simulink library "tqd"  (R2021b)
settings: Solver=VariableStepAuto  StartTime=0.0  StopTime=10.0  RelTol=1e-3
undefined symbols (not defined in the file or in its folder): ATQD_APSDecReq_X_kph, ATQD_APSDecReq_Y_mps2, ATQD_APSDecReqCMD_X_kph, ATQD_APSDecReqTs_X_pct, ATQD_APSDecTimeGain_X_Deg, ATQD_APSDecTimeGain_Y_s, ATQD_APSReqLowSpd_X_Deg, ATQD_AutoHoldReleaseBPS_X_Deg, ATQD_AWDLoadTrqnsGain_X_kg, ATQD_AWDLoadTrqnsGain_Y_pct, ATQD_BOSEnBPSPosn_X_kph, ATQD_BOSMap_X_rpm, ATQD_BOSMap_Y_pct, ATQD_CreepBaseTqD_X_kph, ATQD_CreepBaseTqD_Y_Deg, ATQD_CreepBaseTqR_X_kph, ATQD_CreepBaseTqR_Y_Deg, ATQD_CreepBPSDisPosn_X_Deg, ATQD_CreepBPSDisPosnR_X_Deg, ATQD_CreepBPSEnPosn_X_Deg, ATQD_CreepBPSEnPosnR_X_Deg, ATQD_CreepDeltaTq_X_kph, ATQD_CreepIterm_X_kph, ATQD_CreepIterm_Y_kph, ATQD_CreepItermMaxLimit_X_pct, ATQD_CreepPreloadTime_X_kph, ATQD_CreepPreloadTq_X_kph, ATQD_CreepPreloadTq_Y_s, ATQD_CreepProtTq_X_Deg, ATQD_CreepPterm_X_kph, ATQD_CreepPterm_Y_kph, ATQD_ECOTqMapD_X_rpm, ATQD_ECOTqMapD_Y_pct, ATQD_EOPDTqMapDCon_X_rpm, ATQD_EOPDTqMapDCon_Y_Deg, ATQD_EstInitVehWeight_X_c, ATQD_LHMRollGenMapD_X_rpm, ATQD_LHMRollGenMapD_Y_rpm, ATQD_LHMTqMapD_X_rpm, ATQD_LHMTqMapD_Y_pct, ATQD_NL1TqMapD_X_rpm, ATQD_NL1TqMapD_Y_pct, ATQD_NOPDTqMapDCon_X_rpm, ATQD_NOPDTqMapDCon_Y_Deg, ATQD_NRMRrEDUSpRat_X_rpm, ATQD_NRMRrEDUSpRat_Y_Nm, ATQD_OPDHoldDownRelDelay_X_Deg, ATQD_OPDHoldEnSpd_X_Deg, ATQD_OPDHoldRelDetTime_X_Deg, ATQD_OPDHoldReleaseTq_X_Deg, ATQD_OrigPedTqLowLim_X_Deg, ATQD_OrigPedTqLowLim_Y_pct, ATQD_PedalMapClimbUpLim_X_rpm, ATQD_PedalMapClimbUpLim_Y_Deg, ATQD_PreLoadTq_X_s, ATQD_RollGenMapEL1_X_rpm, ATQD_RollGenMapEL1_Y_rpm, ATQD_SL1TqMapD_X_rpm, ATQD_SL1TqMapD_Y_pct, ATQD_SlideRegenTqGain_X_Gps ... (+491)
libraries: hcu_lib x83, simulink x73, tqr x1
(part 7 of 19)

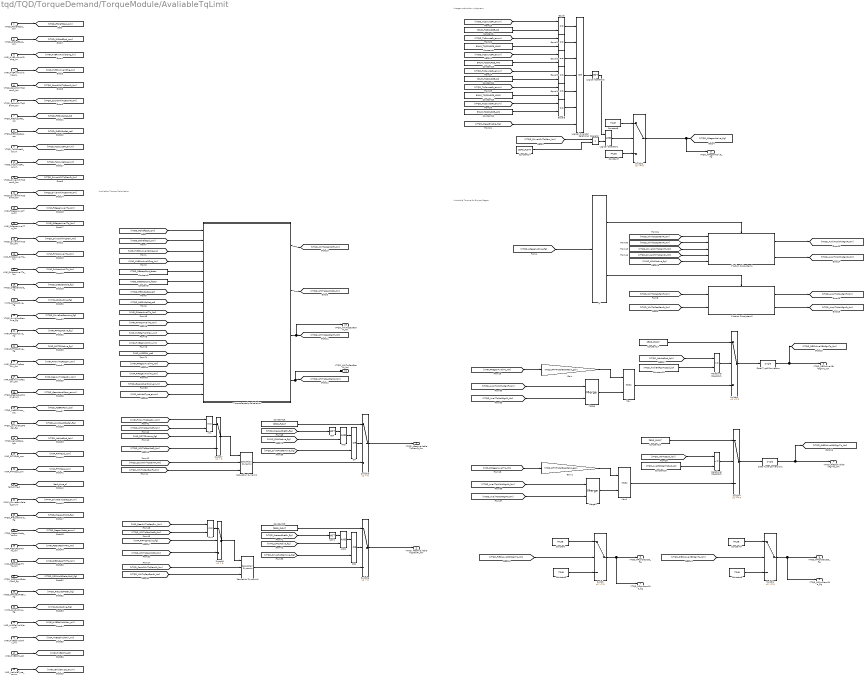
== system tqd/TQD/TorqueDemand/TorqueModule/AvaliableTqLimit ==
  note: Avaiable Torque for B-type Regen
  note: Available Torque Calculation
  note: A-regen activation judgment
  VTQD_FrShaftSpd_rpm : Inport
  VTQD_RrShaftSpd_rpm : Inport  Port=2
  VINP_HVBPwrAvailDchrg_kw : Inport  Port=3
  VINP_HVBPwrAvailChrg_kw : Inport  Port=4
  VTQD_CoordWhlTqDemFr_Nm : Inport  Port=5
  VTQD_CoordWhlTqDemRr_Nm : Inport  Port=6
  VTQD_FrEDUSpRat_rat : Inport  Port=7
  VTQD_RrEDUSpRat_rat : Inport  Port=8
  VTQD_TqSourceFr_enum : Inport  Port=9
  VTQD_TqSourceRr_enum : Inport  Port=10
  VTQD_DriverWhlTqDemFr_Nm : Inport  Port=11
  VTQD_DriverWhlTqDemRr_Nm : Inport  Port=12
  VINP_FrRegenAvailTq_Nm : Inport  Port=13
  VINP_RrRegenAvailTq_Nm : Inport  Port=14
  VTQD_DriverWhlTqDem_Nm : Inport  Port=15
  VINP_FrMotorAvailTq_Nm : Inport  Port=16
  VINP_RrMotorAvailTq_Nm : Inport  Port=17
  VTQD_CreepEnable_flg : Inport  Port=18
  VVMC_ADASActive_flg : Inport  Port=19
  VTQD_DriveProtRemove_flg : Inport  Port=20
  VINP_FrPTCSActive_flg : Inport  Port=21
  VINP_RrPTCSActive_flg : Inport  Port=22
  VINP_FrntAxlTrqReqDrv_Nm : Inport  Port=23
  VINP_RearAxlTrqReqDrv_Nm : Inport  Port=24
  VTQD_GearActualPosn_enum : Inport  Port=25
  VTQD_ActBPSPosn_pct : Inport  Port=26
  VTQD_LowIdleAccPedal_flg : Inport  Port=27
  VTQD_VehActSpd_kph : Inport  Port=28
  VINP_RrTMSpd_rpm : Inport  Port=29
  VINP_FrTMSpd_rpm : Inport  Port=30
  task_time_s : Inport  Port=31
  VPMM_DrivetrainSelect_enum : Inport  Port=32
  VTQD_PreLoadHold_flg : Inport  Port=33
  VTQD_RegenMode_enum : Inport  Port=34
  VINP_FrEDURealTMTq_Nm : Inport  Port=35
  VINP_RrEDURealTMTq_Nm : Inport  Port=36
  VTQD_OPDHoldDelayForP_flg : Inport  Port=37
  VTQD_PreLoadPreEn_flg : Inport  Port=38
  VVMC_CAASActive_flg : Inport  Port=39
  VINP_HVBCellVoltMax_mV : Inport  Port=40
  VINP_HVBCellVoltMin_mV : Inport  Port=41
  VINP_HVBSOH_pct : Inport  Port=42
  VINP_VehicleType_enum : Inport  Port=43
  AND : Logic  AllPortsSameDT=off  OutDataTypeStr=boolean
  AND1 : Logic  AllPortsSameDT=off  OutDataTypeStr=boolean
  Constant : Constant  Value=FALSE
  Constant1 : Constant  Value=ENUM_TQSOURCE_CC
  Constant10 : Constant  Value=ENUM_TQSOURCE_APS
  Constant11 : Constant  Value=ENUM_TQSOURCE_CC
  Constant12 : Constant  Value=ENUM_TQSOURCE_APS
  Constant13 : Constant  Value=ENUM_TQSOURCE_ADAS
  Constant{14,16..17,19..20} (5 alike) : Constant  Value=ZERO_FLOAT
  Constant15 : Constant  Value=KTQD_AvailBrkRgnTqSpd_kph
  Constant18 : Constant  Value=KTQD_AvailBrkRgnTqSpd_kph
  Constant2 : Constant  Value=KTQD_FrBatapCont_factor
  Constant3 : Constant  Value=TRUE
  Constant4 : Constant  Value=FALSE
  Constant5 : Constant  Value=KTQD_RrBatapCont_factor
  Constant6 : Constant  Value=TRUE
  Constant7 : Constant  Value=FALSE
  Constant8 : Constant  Value=TRUE
  Constant9 : Constant  Value=ENUM_TQSOURCE_ADAS
  Data Type Conversion : DataTypeConversion  OutDataTypeStr=single
  Data Type Conversion1 : DataTypeConversion  OutDataTypeStr=single
  Equal{,1..5} (6 alike) : RelationalOperator  Operator===  OutDataTypeStr=boolean  RndMeth=Simplest
  Gain : Gain  Gain=KTQD_FrTMTotalGearRatio_gain
  Gain1 : Gain  Gain=KTQD_RrTMTotalGearRatio_gain
  If : If  IfExpression=u1 ~= 0
  If Action Subsystem1 : Subsystem  TreatAsAtomicUnit=on
  If Action Subsystem2 : Subsystem  TreatAsAtomicUnit=on
  Logical Operator : Logic  Operator=OR  Inputs=7  AllPortsSameDT=off  OutDataTypeStr=boolean
  Logical Operator1 : Logic  AllPortsSameDT=off  OutDataTypeStr=boolean
  Logical Operator2 : Logic  Operator=NOT  AllPortsSameDT=off  OutDataTypeStr=boolean
  Max : MinMax  Function=max  Inputs=2
  Max1 : MinMax  Function=max  Inputs=2
  Merge : Merge
  Merge1 : Merge
  Min : MinMax  Inputs=2
  Min1 : MinMax  Inputs=2
  NOT : Logic  Operator=NOT  AllPortsSameDT=off  OutDataTypeStr=boolean
  NOT1 : Logic  Operator=NOT  AllPortsSameDT=off  OutDataTypeStr=boolean
  OR : Logic  Operator=OR  AllPortsSameDT=off  OutDataTypeStr=boolean
  OR1 : Logic  Operator=OR  AllPortsSameDT=off  OutDataTypeStr=boolean
  Relational Operator : RelationalOperator  Operator=<  OutDataTypeStr=boolean  RndMeth=Simplest
  Relational Operator1 : RelationalOperator  Operator=<=  OutDataTypeStr=boolean  RndMeth=Simplest
  Relational Operator2 : RelationalOperator  Operator=<=  OutDataTypeStr=boolean  RndMeth=Simplest
  Saturation Dynamic : simulink/Discontinuities/Saturation Dynamic  OutMin=[]  OutMax=[]  OutDataTypeStr=Inherit: Same as second input  OutDataType=fixdt(1, 16)  OutScaling=2^-10  DoSatur=off
  Saturation Dynamic1 : simulink/Discontinuities/Saturation Dynamic  OutMin=[]  OutMax=[]  OutDataTypeStr=Inherit: Same as second input  OutDataType=fixdt(1, 16)  OutScaling=2^-10  DoSatur=off
  Switch : Switch
  Switch1 : Switch
  Switch2 : Switch  Criteria=u2 ~= 0
  Switch3 : Switch  Criteria=u2 ~= 0
  Switch4 : Switch  Criteria=u2 ~= 0
  Switch{5..8} (4 alike) : Switch  Criteria=u2 > Threshold
  TorqueCapacityCalcalation : Subsystem
  VTQD_AfterAvailableTqDemFr_Nm : Outport
  VTQD_AfterAvailableTqDemRr_Nm : Outport  Port=2
  VTQD_FrEDUAvailBrkRgnTq_Nm : Outport  Port=3
  VTQD_RrEDUAvailBrkRgnTq_Nm : Outport  Port=4
  VTQD_FrRgnDecrSta_flg : Outport  Port=5
  VTQD_RrRgnDecrSta_flg : Outport  Port=6
  VTQD_FrRgnPermSta_flg : Outport  Port=7
  VTQD_RrRgnPermSta_flg : Outport  Port=8
  VTQD_ARegenActive_flg : Outport  Port=9
  VTQD_WhlTqCapGenFr_Nm : Outport  Port=10
  VTQD_WhlTqCapGenRr_Nm : Outport  Port=11
  wires:
  VINP_FrRegenAvailTq_Nm/1 -> [VINP_FrRegenAvailTq_Nm]
  VINP_RrRegenAvailTq_Nm/1 -> [VINP_RrRegenAvailTq_Nm]
  Merge1/1 -> Max1/2
  [VINP_RrRegenAvailTq_Nm] -> Gain1/1
  Gain1/1 -> Max1/1
  Gain/1 -> Max/1
  Merge/1 -> Max/2
  [VINP_FrRegenAvailTq_Nm] -> Gain/1
  [VTQD_ARegenActive_flg] -> If/1
  Switch1/1 -> VTQD_RrRgnDecrSta_flg/1, VTQD_RrRgnPermSta_flg/1
  Constant6/1 -> Switch1/3
  Constant4/1 -> Switch1/1
  [VTQD_RrEDUAvailBrkRgnTq_Nm] -> Switch1/2
  Switch/1 -> VTQD_FrRgnDecrSta_flg/1, VTQD_FrRgnPermSta_flg/1
  Constant3/1 -> Switch/3
  Constant/1 -> Switch/1
  [VTQD_FrEDUAvailBrkRgnTq_Nm] -> Switch/2
  If/2 -> If Action Subsystem2/Action
  If/1 -> If Action Subsystem1/Action
  Data Type Conversion1/1 -> VTQD_RrEDUAvailBrkRgnTq_Nm/1, [VTQD_RrEDUAvailBrkRgnTq_Nm]  "VTQD_RrEDUAvailBrkRgnTq_Nm"
  Data Type Conversion/1 -> VTQD_FrEDUAvailBrkRgnTq_Nm/1, [VTQD_FrEDUAvailBrkRgnTq_Nm]  "VTQD_FrEDUAvailBrkRgnTq_Nm"
  TorqueCapacityCalcalation/4(VTQD_WhlTqCapGenRr_Nm) -> VTQD_WhlTqCapGenRr_Nm/1, [VTQD_WhlTqCapGenRr_Nm]
  TorqueCapacityCalcalation/2(VTQD_WhlTqCapMotRr_Nm) -> [VTQD_WhlTqCapMotRr_Nm]
  VTQD_RrShaftSpd_rpm/1 -> [VTQD_RrShaftSpd_rpm]
  [VTQD_RrEDUSpRat_rat] -> TorqueCapacityCalcalation/8(VTQD_RrEDUSpRat_rat)
  [VTQD_FrEDUSpRat_rat] -> TorqueCapacityCalcalation/7(VTQD_FrEDUSpRat_cmd)
  Constant5/1 -> TorqueCapacityCalcalation/6(KTQD_RrBatapCont_factor)
  [VTQD_RrShaftSpd_rpm] -> TorqueCapacityCalcalation/2(VTQD_RrShaftSpd_rpm)
  Constant2/1 -> TorqueCapacityCalcalation/5(KTQD_FrBatapCont_factor)
  [VINP_HVBPwrAvailChrg_kw] -> TorqueCapacityCalcalation/4(VINP_HVBPwrAvailChrg_kw)
  [VINP_HVBPwrAvailDchrg_kw] -> TorqueCapacityCalcalation/3(VINP_HVBPwrAvailDchrg_kw)
  [VTQD_FrShaftSpd_rpm] -> TorqueCapacityCalcalation/1(VTQD_FrShaftSpd_rpm)
  TorqueCapacityCalcalation/1(VTQD_WhlTqCapMotFr_Nm) -> [VTQD_WhlTqCapMotFr_Nm]
  TorqueCapacityCalcalation/3(VTQD_WhlTqCapGenFr_Nm) -> VTQD_WhlTqCapGenFr_Nm/1, [VTQD_WhlTqCapGenFr_Nm]
  If Action Subsystem2/2(VTQD_AvailTqNoARgnRr_Nm) -> [VTQD_AvailTqNoARgnRr_Nm]
  If Action Subsystem2/1(VTQD_AvailTqNoARgnFr_Nm) -> [VTQD_AvailTqNoARgnFr_Nm]
  [VTQD_WhlTqCapGenRr_Nm] -> If Action Subsystem2/2(VTQD_WhlTqCapGenR_Nm)
  [VTQD_WhlTqCapGenFr_Nm] -> If Action Subsystem2/1(VTQD_WhlTqCapGenF_Nm)
  [VTQD_WhlTqCapGenRr_Nm] -> If Action Subsystem1/2(VTQD_WhlTqCapGenR_Nm)
  [VTQD_WhlTqCapGenFr_Nm] -> If Action Subsystem1/1(VTQD_WhlTqCapGenF_Nm)
  [VTQD_DriverWhlTqDemRr_Nm] -> If Action Subsystem1/4(VTQD_DriverWhlTqDemRr_Nm)
  [VTQD_DriverWhlTqDemFr_Nm] -> If Action Subsystem1/3(VTQD_DriverWhlTqDemFr_Nm)
  VTQD_DriverWhlTqDemRr_Nm/1 -> [VTQD_DriverWhlTqDemRr_Nm]
  VTQD_DriverWhlTqDemFr_Nm/1 -> [VTQD_DriverWhlTqDemFr_Nm]
  VTQD_TqSourceFr_enum/1 -> [VTQD_TqSourceFr_enum]
  VTQD_RrEDUSpRat_rat/1 -> [VTQD_RrEDUSpRat_rat]
  VTQD_FrEDUSpRat_rat/1 -> [VTQD_FrEDUSpRat_rat]
  VTQD_CoordWhlTqDemRr_Nm/1 -> [VTQD_CoordWhlTqDemRr_Nm]
  VTQD_CoordWhlTqDemFr_Nm/1 -> [VTQD_CoordWhlTqDemFr_Nm]
  VINP_HVBPwrAvailDchrg_kw/1 -> [VINP_HVBPwrAvailDchrg_kw]
  VTQD_FrShaftSpd_rpm/1 -> [VTQD_FrShaftSpd_rpm]
  VINP_HVBPwrAvailChrg_kw/1 -> [VINP_HVBPwrAvailChrg_kw]
  VTQD_TqSourceRr_enum/1 -> [VTQD_TqSourceRr_enum]
  Switch2/1 -> [VTQD_ARegenActive_flg], VTQD_ARegenActive_flg/1  "VTQD_ARegenActive_flg"
  VTQD_DriverWhlTqDem_Nm/1 -> [VTQD_DriverWhlTqDem_Nm]
  VINP_RrMotorAvailTq_Nm/1 -> [VINP_RrMotorAvailTq_Nm]
  VINP_FrMotorAvailTq_Nm/1 -> [VINP_FrMotorAvailTq_Nm]
  [VINP_FrMotorAvailTq_Nm] -> TorqueCapacityCalcalation/9(VINP_FrMotorAvailTq_Nm)
  [VINP_RrMotorAvailTq_Nm] -> TorqueCapacityCalcalation/10(VINP_RrMotorAvailTq_Nm)
  VTQD_CreepEnable_flg/1 -> [VTQD_CreepEnable_flg]
  [VTQD_TqSourceFr_enum] -> Equal/1
  Constant1/1 -> Equal/2
  Constant9/1 -> Equal1/2
  [VTQD_TqSourceFr_enum] -> Equal1/1
  [VTQD_TqSourceFr_enum] -> Equal2/1
  Constant10/1 -> Equal2/2
  Constant12/1 -> Equal5/2
  [VTQD_TqSourceRr_enum] -> Equal5/1
  [VTQD_TqSourceRr_enum] -> Equal4/1
  Constant13/1 -> Equal4/2
  Constant11/1 -> Equal3/2
  [VTQD_TqSourceRr_enum] -> Equal3/1
  Equal5/1 -> Logical Operator/6
  Equal4/1 -> Logical Operator/5
  Equal3/1 -> Logical Operator/4
  Equal2/1 -> Logical Operator/3
  Equal1/1 -> Logical Operator/2
  Equal/1 -> Logical Operator/1
  [VTQD_CreepEnable_flg] -> Logical Operator/7
  Logical Operator/1 -> Logical Operator2/1
  Logical Operator1/1 -> Switch2/2
  [VTQD_DriverWhlTqDem_Nm] -> Relational Operator/1
  Relational Operator/1 -> Logical Operator1/2
  Constant14/1 -> Relational Operator/2
  Constant7/1 -> Switch2/3
  Constant8/1 -> Switch2/1
  Logical Operator2/1 -> Logical Operator1/1
  Constant17/1 -> Switch3/1
  Relational Operator1/1 -> Switch3/2
  Constant15/1 -> Relational Operator1/2
  Max/1 -> Switch3/3
  Switch3/1 -> Data Type Conversion/1
  Constant20/1 -> Switch4/1
  Max1/1 -> Switch4/3
  Relational Operator2/1 -> Switch4/2
  Constant18/1 -> Relational Operator2/2
  Switch4/1 -> Data Type Conversion1/1
  VVMC_ADASActive_flg/1 -> [VVMC_ADASActive_flg]
  [VVMC_ADASActive_flg] -> If Action Subsystem1/5(VVMC_ADASActive_flg)
  [VTQD_AvailTqNoARgnRr_Nm] -> Merge1/2
  [VTQD_AvailTqWithARgnRr_Nm] -> Merge1/1
  [VTQD_AvailTqNoARgnFr_Nm] -> Merge/2
  [VTQD_AvailTqWithARgnFr_Nm] -> Merge/1
  Constant16/1 -> Switch5/1
  Switch5/1 -> VTQD_AfterAvailableTqDemFr_Nm/1  "VTQD_AfterAvailableTqDemFr_Nm"
  Saturation Dynamic/1 -> Switch5/3
  Constant19/1 -> Switch6/1
  Saturation Dynamic1/1 -> Switch6/3
  Switch6/1 -> VTQD_AfterAvailableTqDemRr_Nm/1  "VTQD_AfterAvailableTqDemRr_Nm"
  VTQD_DriveProtRemove_flg/1 -> [VTQD_DriveProtRemove_flg]
  [VTQD_CoordWhlTqDemFr_Nm] -> Saturation Dynamic/2
  Switch7/1 -> Saturation Dynamic/1  "VTQD_FrAvailableTqUpLimt_Nm"
  [VTQD_WhlTqCapMotFr_Nm] -> Switch7/3
  [VINP_FrPTCSActive_flg] -> Switch7/2
  VINP_RearAxlTrqReqDrv_Nm/1 -> [VINP_RearAxlTrqReqDrv_Nm]
  VINP_FrntAxlTrqReqDrv_Nm/1 -> [VINP_FrntAxlTrqReqDrv_Nm]
  VINP_RrPTCSActive_flg/1 -> [VINP_RrPTCSActive_flg]
  VINP_FrPTCSActive_flg/1 -> [VINP_FrPTCSActive_flg]
  [VINP_RrPTCSActive_flg] -> Switch8/2
  [VTQD_WhlTqCapMotRr_Nm] -> Switch8/3
  Switch8/1 -> Saturation Dynamic1/1  "VTQD_RrAvailableTqUpLimt_Nm"
  [VTQD_CoordWhlTqDemRr_Nm] -> Saturation Dynamic1/2
  [VTQD_WhlTqCapMotFr_Nm] -> Min/2
  Min/1 -> Switch7/1
  [VINP_FrntAxlTrqReqDrv_Nm] -> Min/1
  [VTQD_WhlTqCapMotRr_Nm] -> Min1/2
  Min1/1 -> Switch8/1
  [VINP_RearAxlTrqReqDrv_Nm] -> Min1/1
  VTQD_GearActualPosn_enum/1 -> [VTQD_GearActualPosn_enum]
  VTQD_ActBPSPosn_pct/1 -> [VTQD_ActBPSPosn_pct]
  VTQD_LowIdleAccPedal_flg/1 -> [VTQD_LowIdleAccPedal_flg]
  VTQD_VehActSpd_kph/1 -> [VTQD_VehActSpd_kph]
  VINP_RrTMSpd_rpm/1 -> [VINP_RrTMSpd_rpm]
  VINP_FrTMSpd_rpm/1 -> [VINP_FrTMSpd_rpm]
  task_time_s/1 -> [task_time_s]
  VPMM_DrivetrainSelect_enum/1 -> [VPMM_DrivetrainSelect_enum]
  [VTQD_VehActSpd_kph] -> Relational Operator1/1
  [VTQD_VehActSpd_kph] -> Relational Operator2/1
  [VTQD_WhlTqCapGenFr_Nm] -> Saturation Dynamic/3
  [VTQD_WhlTqCapGenRr_Nm] -> Saturation Dynamic1/3
  VTQD_PreLoadHold_flg/1 -> [VTQD_PreLoadHold_flg]
  VTQD_RegenMode_enum/1 -> [VTQD_RegenMode_enum]
  VINP_RrEDURealTMTq_Nm/1 -> [VINP_RrEDURealTMTq_Nm]
  VINP_FrEDURealTMTq_Nm/1 -> [VINP_FrEDURealTMTq_Nm]
  VTQD_OPDHoldDelayForP_flg/1 -> [VTQD_OPDHoldDelayForP_flg]
  VVMC_CAASActive_flg/1 -> [VVMC_CAASActive_flg]
  VTQD_PreLoadPreEn_flg/1 -> [VTQD_PreLoadPreEn_flg]
  OR/1 -> Switch5/2
  AND/1 -> OR/1
  [VTQD_DriveProtRemove_flg] -> OR/2
  NOT/1 -> AND/1
  [VTQD_PreLoadPreEn_flg] -> NOT/1
  [VVMC_CAASActive_flg] -> AND/2
  NOT1/1 -> AND1/1
  AND1/1 -> OR1/1
  [VVMC_CAASActive_flg] -> AND1/2
  [VTQD_PreLoadPreEn_flg] -> NOT1/1
  [VTQD_DriveProtRemove_flg] -> OR1/2
  OR1/1 -> Switch6/2
  VINP_HVBCellVoltMin_mV/1 -> [VINP_HVBCellVoltMin_mV]
  VINP_HVBSOH_pct/1 -> [VINP_HVBSOH_pct]
  VINP_HVBCellVoltMax_mV/1 -> [VINP_HVBCellVoltMax_mV]
  [VINP_HVBCellVoltMax_mV] -> TorqueCapacityCalcalation/11(VINP_HVBCellVoltMax_mV)
  [VINP_HVBCellVoltMin_mV] -> TorqueCapacityCalcalation/12(VINP_HVBCellVoltMin_mV)
  [VINP_HVBSOH_pct] -> TorqueCapacityCalcalation/13(VINP_HVBSOH_pct)
  If Action Subsystem1/1(VTQD_AvailTqWithARgnFr_Nm) -> [VTQD_AvailTqWithARgnFr_Nm]
  If Action Subsystem1/2(VTQD_AvailTqWithARgnRr_Nm) -> [VTQD_AvailTqWithARgnRr_Nm]
  [VINP_RrRegenAvailTq_Nm] -> TorqueCapacityCalcalation/15(VINP_RrRegenAvailTq_Nm)
  [VINP_FrRegenAvailTq_Nm] -> TorqueCapacityCalcalation/14(VINP_FrRegenAvailTq_Nm)
  [VTQD_GearActualPosn_enum] -> TorqueCapacityCalcalation/16(VTQD_GearActualPosn_enum)
  VINP_VehicleType_enum/1 -> [VINP_VehicleType_enum]
  [VINP_VehicleType_enum] -> TorqueCapacityCalcalation/17(VINP_VehicleType_enum)

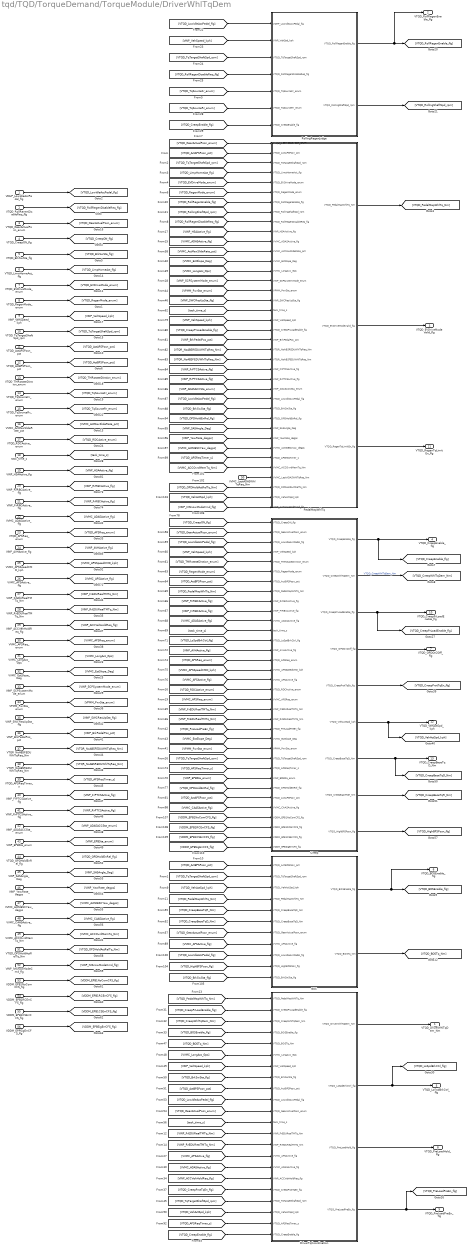
== system tqd/TQD/TorqueDemand/TorqueModule/DriverWhlTqDem ==
  VDHP_LowIdleAccPedal_flg : Inport
  VTQD_RollRegenDisableReq_flg : Inport  Port=2
  VTQD_GearActualPosn_enum : Inport  Port=3
  "VTQD_CreepON_flg " : Inport  Port=4
  VTQD_BrkSwSta_flg : Inport  Port=5
  VTQD_LimpHomeAct_flg : Inport  Port=6
  VTQD_EVDriveMode_enum : Inport  Port=7
  VTQD_RegenMode_enum : Inport  Port=8
  VINP_VehSpeed_kph : Inport  Port=9
  VTQD_TqTargetShaftSpd_rpm : Inport  Port=10
  VTQD_ActAPSPosn_pct : Inport  Port=11
  VTQD_ActBPSPosn_pct : Inport  Port=12
  VTQD_TMRotateDirction_enum : Inport  Port=13
  VTQD_TqSourceFr_enum : Inport  Port=14
  VTQD_TqSourceRr_enum : Inport  Port=15
  VVMC_ActMaxSlideRate_pct : Inport  Port=16
  VTQD_RDCActive_enum : Inport  Port=17
  task_time_s : Inport  Port=18
  VINP_HSAActive_flg : Inport  Port=19
  VINP_RrRBCActive_flg : Inport  Port=20
  VINP_FrRBCActive_flg : Inport  Port=21
  VVMC_ADASActive_flg : Inport  Port=22
  VTQD_APSReq_enum : Inport  Port=23
  VINP_AVHActive_flg : Inport  Port=24
  VVMC_APSSpeedCMD_kph : Inport  Port=25
  VVMC_APSActive_flg : Inport  Port=26
  VINP_FrEDURealTMTq_Nm : Inport  Port=27
  VINP_RrEDURealTMTq_Nm : Inport  Port=28
  VINP_ACCVehHoldReq_flg : Inport  Port=29
  VVMC_APSReq_enum : Inport  Port=30
  VVMC_LongAcc_Gps : Inport  Port=31
  VVMC_EstSlope_Deg : Inport  Port=32
  VINP_SCPSystemMode_enum : Inport  Port=33
  VPMM_PwrSta_enum : Inport  Port=34
  VINP_SWCResUpSta_flg : Inport  Port=35
  VINP_BrkPedalPos_pct : Inport  Port=36
  VTQR_NoABSFEDUWhlTqReq_Nm : Inport  Port=37
  VTQR_NoABSREDUWhlTqReq_Nm : Inport  Port=38
  VTQD_APSReqTimer_s : Inport  Port=39
  VINP_FrPTCSActive_flg : Inport  Port=40
  VINP_RrPTCSActive_flg : Inport  Port=41
  VINP_ADASACCSta_enum : Inport  Port=42
  VINP_EPBSta_enum : Inport  Port=43
  VTQD_OPDHoldEnRel_flg : Inport  Port=44
  VINP_SASAngle_Deg : Inport  Port=45
  VINP_YawRate_degps : Inport  Port=46
  VVMC_ActStESCYaw_degps : Inport  Port=47
  VVMC_CAASActive_flg : Inport  Port=48
  VVMC_ACCOvrdMemTq_Nm : Inport  Port=49
  VVMC_LastADASWhlTqReq_Nm : Inport  Port=50
  VTQD_OPDHoldActRelTq_Nm : Inport  Port=51
  VINP_IVISnowModeCmd_flg : Inport  Port=52
  VDDM_EPB1NoComCFS_flg : Inport  Port=53
  VDDM_EPB1RCErrCFS_flg : Inport  Port=54
  VDDM_EPB1CSErrCFS_flg : Inport  Port=55
  VDDM_EPBSigErrCFS_flg : Inport  Port=56
  BOS : Subsystem
  Creep : Subsystem
  DriverTqCoordination : Subsystem
  PedalMapWhlTq : Subsystem
  RollingRegenJudge : Subsystem
  VTQD_DriverWhlTqDem_Nm : Outport
  VTQD_RollRegenEnable_flg : Outport  Port=2
  VTQD_EVDriveModeValid_flg : Outport  Port=3
  VTQD_CreepEnable_flg : Outport  Port=4
  VTQD_LoSpdBrkCtrl_flg : Outport  Port=5
  VTQD_BOSEnable_flg : Outport  Port=6
  VTQD_OPDOn2Off_flg : Outport  Port=7
  VTQD_PreLoadHold_flg : Outport  Port=8
  VTQD_PreLoadPreEn_flg : Outport  Port=9
  VTQD_CreepPrLoadEnable_flg : Outport  Port=10
  VTQD_RegenTqLimitEn_flg : Outport  Port=11
  VTQD_VehActSpd_kph : Outport  Port=12
  VTQD_CreepBaseTqD_Nm : Outport  Port=13
  wires:
  VTQD_BrkSwSta_flg/1 -> [VTQD_BrkSwSta_flg]
  VTQD_ActBPSPosn_pct/1 -> [VTQD_ActBPSPosn_pct]
  VTQD_RegenMode_enum/1 -> [VTQD_RegenMode_enum]
  VINP_VehSpeed_kph/1 -> [VINP_VehSpeed_kph]
  "VTQD_CreepON_flg "/1 -> [VTQD_CreepON_flg]
  PedalMapWhlTq/1(VTQD_PedalMapWhlTq_Nm) -> [VTQD_PedalMapWhlTq_Nm]
  VTQD_LimpHomeAct_flg/1 -> [VTQD_LimpHomeAct_flg]
  VTQD_TqTargetShaftSpd_rpm/1 -> [VTQD_TqTargetShaftSpd_rpm]
  VTQD_EVDriveMode_enum/1 -> [VTQD_EVDriveMode_enum]
  VTQD_ActAPSPosn_pct/1 -> [VTQD_ActAPSPosn_pct]
  VTQD_GearActualPosn_enum/1 -> [VTQD_GearActualPosn_enum]
  VDHP_LowIdleAccPedal_flg/1 -> [VTQD_LowIdleAccPedal_flg]
  BOS/2(VTQD_BOSTq_Nm) -> [VTQD_BOSTq_Nm]
  BOS/1(VTQD_BOSEnable_flg) -> [VTQD_BOSEnable_flg], VTQD_BOSEnable_flg/1
  [VTQD_ActBPSPosn_pct] -> BOS/1(VTQD_ActBPSPosn_pct)
  [VTQD_TqTargetShaftSpd_rpm] -> BOS/2(VTQD_TqTargetShaftSpd_rpm)
  RollingRegenJudge/1(VTQD_RollRegenEnable_flg) -> VTQD_RollRegenEnable_flg/1, [VTQD_RollRegenEnable_flg]
  RollingRegenJudge/2(VTQD_RollingShaftSpd_rpm) -> [VTQD_RollingShaftSpd_rpm]
  VTQD_RollRegenDisableReq_flg/1 -> [VTQD_RollRegenDisableReq_flg]
  PedalMapWhlTq/2(VTQD_EVDriveModeValid_flg) -> VTQD_EVDriveModeValid_flg/1
  VTQD_TMRotateDirction_enum/1 -> [VTQD_TMRotateDirction_enum]
  [VTQD_GearActualPosn_enum] -> PedalMapWhlTq/1(VTQD_GearActualPosn_enum)
  [VTQD_LimpHomeAct_flg] -> PedalMapWhlTq/4(VTQD_LimpHomeAct_flg)
  [VTQD_ActAPSPosn_pct] -> PedalMapWhlTq/2(VTQD_ActAPSPosn_pct)
  [VTQD_TqTargetShaftSpd_rpm] -> PedalMapWhlTq/3(VTQD_TqTargetShaftSpd_rpm)
  [VTQD_RollRegenEnable_flg] -> PedalMapWhlTq/7(VTQD_RollRegenEnable_flg)
  [VTQD_RollingShaftSpd_rpm] -> PedalMapWhlTq/8(VTQD_RollingShaftSpd_rpm)
  [VTQD_RegenMode_enum] -> PedalMapWhlTq/6(VTQD_RegenMode_enum)
  [VTQD_EVDriveMode_enum] -> PedalMapWhlTq/5(VTQD_EVDriveMode_enum)
  [VTQD_TqSourceRr_enum] -> RollingRegenJudge/6(VTQD_TqSourceRr_enum)
  [VINP_VehSpeed_kph] -> RollingRegenJudge/2(VINP_VehSpd_kph)
  [VTQD_TqTargetShaftSpd_rpm] -> RollingRegenJudge/3(VTQD_TqTargetShaftSpd_rpm)
  [VTQD_TqSourceFr_enum] -> RollingRegenJudge/5(VTQD_TqSourceFr_enum)
  [VTQD_CreepEnable_flg] -> RollingRegenJudge/7(VTQD_CreepEnable_flg)
  [VTQD_LowIdleAccPedal_flg] -> RollingRegenJudge/1(VDHP_LowIdleAccPedal_flg)
  VTQD_TqSourceFr_enum/1 -> [VTQD_TqSourceFr_enum]
  VTQD_TqSourceRr_enum/1 -> [VTQD_TqSourceRr_enum]
  VVMC_ActMaxSlideRate_pct/1 -> [VVMC_ActMaxSlideRate_pct]
  VTQD_RDCActive_enum/1 -> [VTQD_RDCActive_enum]
  task_time_s/1 -> [task_time_s]
  [VTQD_RollRegenDisableReq_flg] -> RollingRegenJudge/4(VTQD_RollRegenDisableReq_flg)
  [VINP_VehSpeed_kph] -> DriverTqCoordination/7(VINP_VehSpeed_kph)
  [task_time_s] -> DriverTqCoordination/12(task_time_s)
  [VTQD_LowIdleAccPedal_flg] -> DriverTqCoordination/10(VTQD_LowIdleAccPedal_flg)
  [VTQD_GearActualPosn_enum] -> DriverTqCoordination/11(VTQD_GearActualPosn_enum)
  [VTQD_CreepPrLoadEnable_flg] -> DriverTqCoordination/2(VTQD_CreepPrLoadEnable_flg)
  [VTQD_PedalMapWhlTq_Nm] -> DriverTqCoordination/1(VTQD_PedalMapWhlTq_Nm)
  [VTQD_ActBPSPosn_pct] -> DriverTqCoordination/9(VTQD_ActBPSPosn_pct)
  [VTQD_BOSEnable_flg] -> DriverTqCoordination/4(VTQD_BOSEnable_flg)
  [VTQD_CreepWhlTqDem_Nm] -> DriverTqCoordination/3(VTQD_CreepWhlTqDem_Nm)
  [VTQD_BrkSwSta_flg] -> DriverTqCoordination/8(VTQD_BrkSwSta_flg)
  DriverTqCoordination/2(VTQD_LoSpdBrkCtrl_flg) -> [VTQD_LoSpdBrkCtrl_flg], VTQD_LoSpdBrkCtrl_flg/1
  DriverTqCoordination/1(VTQD_DriverWhlTqDem_Nm) -> VTQD_DriverWhlTqDem_Nm/1
  [VINP_RrRBCActive_flg] -> Creep/9(VINP_RrRBCActive_flg)
  [VINP_FrRBCActive_flg] -> Creep/10(VINP_FrRBCActive_flg)
  [VINP_VehSpeed_kph] -> Creep/4(VINP_VehSpeed_kph)
  [VTQD_ActBPSPosn_pct] -> Creep/7(VTQD_ActBPSPosn_pct)
  [VTQD_TMRotateDirction_enum] -> Creep/5(VTQD_TMRotateDirction_enum)
  [VTQD_CreepON_flg] -> Creep/1(VTQD_CreepON_flg)
  [VTQD_LowIdleAccPedal_flg] -> Creep/3(VTQD_LowIdleAccPedal_flg)
  [VTQD_APSReq_enum] -> Creep/15(VTQD_APSReq_enum)
  [VVMC_APSActive_flg] -> Creep/17(VVMC_APSActive_flg)
  [VTQD_RegenMode_enum] -> Creep/6(VTQD_RegenMode_enum)
  [VINP_AVHActive_flg] -> Creep/14(VINP_AVHActive_flg)
  [VVMC_APSSpeedCMD_kph] -> Creep/16(VVMC_APSSpeedCMD_kph)
  [VTQD_PedalMapWhlTq_Nm] -> Creep/8(VTQD_PedalMapWhlTq_Nm)
  [VTQD_GearActualPosn_enum] -> Creep/2(VTQD_GearActualPosn_enum)
  [VVMC_ADASActive_flg] -> Creep/11(VVMC_ADASActive_flg)
  [task_time_s] -> Creep/12(task_time_s)
  [VTQD_LoSpdBrkCtrl_flg] -> Creep/13(VTQD_LoSpdBrkCtrl_flg)
  Creep/1(VTQD_CreepEnable_flg) -> [VTQD_CreepEnable_flg], VTQD_CreepEnable_flg/1
  Creep/2(VTQD_CreepWhlTqDem_Nm) -> [VTQD_CreepWhlTqDem_Nm]  "VTQD_CreepWhlTqDem_Nm"
  Creep/3(VTQD_CreepPrLoadEnable_flg) -> VTQD_CreepPrLoadEnable_flg/1, [VTQD_CreepPrLoadEnable_flg]
  VVMC_APSActive_flg/1 -> [VVMC_APSActive_flg]
  VTQD_APSReq_enum/1 -> [VTQD_APSReq_enum]
  VVMC_ADASActive_flg/1 -> [VVMC_ADASActive_flg]
  VINP_AVHActive_flg/1 -> [VINP_AVHActive_flg]
  VVMC_APSSpeedCMD_kph/1 -> [VVMC_APSSpeedCMD_kph]
  VINP_FrRBCActive_flg/1 -> [VINP_FrRBCActive_flg]
  VINP_RrRBCActive_flg/1 -> [VINP_RrRBCActive_flg]
  VINP_HSAActive_flg/1 -> [VINP_HSAActive_flg]
  [VTQD_RollRegenDisableReq_flg] -> PedalMapWhlTq/9(VTQD_RollRegenDisableReq_flg)
  [VINP_HSAActive_flg] -> PedalMapWhlTq/10(VINP_HSAActive_flg)
  Creep/4(VTQD_OPDOn2Off_flg) -> VTQD_OPDOn2Off_flg/1
  VINP_RrEDURealTMTq_Nm/1 -> [VINP_RrEDURealTMTq_Nm]
  VINP_FrEDURealTMTq_Nm/1 -> [VINP_FrEDURealTMTq_Nm]
  [VINP_FrEDURealTMTq_Nm] -> DriverTqCoordination/13(VINP_FrEDURealTMTq_Nm)
  [VINP_RrEDURealTMTq_Nm] -> DriverTqCoordination/14(VINP_RrEDURealTMTq_Nm)
  DriverTqCoordination/3(VTQD_PreLoadHold_flg) -> VTQD_PreLoadHold_flg/1
  [VVMC_ADASActive_flg] -> PedalMapWhlTq/11(VVMC_ADASActive_flg)
  [VTQD_RDCActive_enum] -> Creep/18(VTQD_RDCActive_enum)
  VINP_ACCVehHoldReq_flg/1 -> [VINP_ACCVehHoldReq_flg]
  VVMC_APSReq_enum/1 -> [VVMC_APSReq_enum]
  [VVMC_APSReq_enum] -> Creep/19(VVMC_APSReq_enum)
  [VVMC_APSActive_flg] -> DriverTqCoordination/15(VVMC_APSActive_flg)
  [VVMC_ADASActive_flg] -> DriverTqCoordination/16(VVMC_ADASActive_flg)
  [VINP_ACCVehHoldReq_flg] -> DriverTqCoordination/17(VINP_ACCVehHoldReq_flg)
  [VINP_RrEDURealTMTq_Nm] -> Creep/21(VINP_RrEDURealTMTq_Nm)
  [VINP_FrEDURealTMTq_Nm] -> Creep/20(" VINP_FrEDURealTMTq_Nm")
  Creep/5(VTQD_CreepProtTqEn_flg) -> [VTQD_CreepProtTqEn_flg]
  [VTQD_CreepProtTqEn_flg] -> DriverTqCoordination/18(VTQD_CreepProtTqEn_flg)
  [VVMC_ActMaxSlideRate_pct] -> PedalMapWhlTq/12(VVMC_ActMaxSlideRate_pct)
  VVMC_LongAcc_Gps/1 -> [VVMC_LongAcc_Gps]
  VVMC_EstSlope_Deg/1 -> [VVMC_EstSlope_Deg]
  [VVMC_LongAcc_Gps] -> PedalMapWhlTq/14(VVMC_LongAcc_Gps)
  [VVMC_EstSlope_Deg] -> PedalMapWhlTq/13(VVMC_EstSlope_Deg)
  PedalMapWhlTq/3(VTQD_RegenTqLimitEn_flg) -> VTQD_RegenTqLimitEn_flg/1
  DriverTqCoordination/4(VTQD_PreLoadPreEn_flg) -> [VTQD_PreLoadPreEn_flg], VTQD_PreLoadPreEn_flg/1
  [VTQD_PreLoadPreEn_flg] -> Creep/22(VTQD_PreLoadPreEn_flg)
  [VVMC_EstSlope_Deg] -> Creep/23(VVMC_EstSlope_Deg)
  [VPMM_PwrSta_enum] -> Creep/24(VPMM_PwrSta_enum)
  [VTQD_TqTargetShaftSpd_rpm] -> DriverTqCoordination/19(VTQD_TqTargetShaftSpd_rpm)
  [VINP_SCPSystemMode_enum] -> PedalMapWhlTq/15(VINP_SCPSystemMode_enum)
  [VPMM_PwrSta_enum] -> PedalMapWhlTq/16(VPMM_PwrSta_enum)
  [VINP_SWCResUpSta_flg] -> PedalMapWhlTq/17(VINP_SWCResUpSta_flg)
  [task_time_s] -> PedalMapWhlTq/18(task_time_s)
  [VINP_VehSpeed_kph] -> PedalMapWhlTq/19(VINP_VehSpeed_kph)
  [VTQD_CreepPrLoadEnable_flg] -> PedalMapWhlTq/20(VTQD_CreepPrLoadEnable_flg)
  [VINP_BrkPedalPos_pct] -> PedalMapWhlTq/21(VINP_BrkPedalPos_pct)
  [VTQR_NoABSREDUWhlTqReq_Nm] -> PedalMapWhlTq/22(VTQR_NoABSREDUWhlTqReq_Nm)
  [VTQR_NoABSFEDUWhlTqReq_Nm] -> PedalMapWhlTq/23(VTQR_NoABSFEDUWhlTqReq_Nm)
  [VINP_FrPTCSActive_flg] -> PedalMapWhlTq/24(VINP_FrPTCSActive_flg)
  [VINP_RrPTCSActive_flg] -> PedalMapWhlTq/25(VINP_RrPTCSActive_flg)
  [VINP_ADASACCSta_enum] -> PedalMapWhlTq/26(VINP_ADASACCSta_enum)
  [VTQD_LowIdleAccPedal_flg] -> PedalMapWhlTq/27(VTQD_LowIdleAccPedal_flg)
  [VTQD_BrkSwSta_flg] -> PedalMapWhlTq/28(VTQD_BrkSwSta_flg)
  [VTQD_TqTargetShaftSpd_rpm] -> Creep/25(VTQD_TqTargetShaftSpd_rpm)
  [VTQD_APSReqTimer_s] -> Creep/26(VTQD_APSReqTimer_s)
  [VINP_EPBSta_enum] -> Creep/27(VINP_EPBSta_enum)
  Creep/6(VTQD_VehActSpd_kph) -> [VTQD_VehActSpd_kph], VTQD_VehActSpd_kph/1
  VINP_EPBSta_enum/1 -> [VINP_EPBSta_enum]
  VINP_RrPTCSActive_flg/1 -> [VINP_RrPTCSActive_flg]
  VINP_SCPSystemMode_enum/1 -> [VINP_SCPSystemMode_enum]
  VINP_BrkPedalPos_pct/1 -> [VINP_BrkPedalPos_pct]
  VINP_FrPTCSActive_flg/1 -> [VINP_FrPTCSActive_flg]
  VTQD_APSReqTimer_s/1 -> [VTQD_APSReqTimer_s]
  VTQR_NoABSFEDUWhlTqReq_Nm/1 -> [VTQR_NoABSFEDUWhlTqReq_Nm]
  VINP_ADASACCSta_enum/1 -> [VINP_ADASACCSta_enum]
  VTQR_NoABSREDUWhlTqReq_Nm/1 -> [VTQR_NoABSREDUWhlTqReq_Nm]
  VINP_SWCResUpSta_flg/1 -> [VINP_SWCResUpSta_flg]
  VPMM_PwrSta_enum/1 -> [VPMM_PwrSta_enum]
  [VTQD_PedalMapWhlTq_Nm] -> BOS/4(VTQD_PedalMapWhlTq_Nm)
  [VTQD_VehActSpd_kph] -> BOS/3(VTQD_VehActSpd_kph)
  Creep/7(VTQD_CreepBaseTqD_Nm) -> [VTQD_CreepBaseTqD_Nm], VTQD_CreepBaseTqD_Nm/1
  Creep/8(VTQD_CreepBaseTqR_Nm) -> [VTQD_CreepBaseTqR_Nm]
  [VTQD_BOSTq_Nm] -> DriverTqCoordination/5(VTQD_BOSTq_Nm)
  [VTQD_CreepBaseTqR_Nm] -> BOS/5(VTQD_CreepBaseTqR_Nm)
  [VTQD_CreepBaseTqD_Nm] -> BOS/6(VTQD_CreepBaseTqD_Nm)
  [VTQD_GearActualPosn_enum] -> BOS/7(VTQD_GearActualPosn_enum)
  VTQD_OPDHoldEnRel_flg/1 -> [VTQD_OPDHoldEnRel_flg]
  [VTQD_OPDHoldEnRel_flg] -> Creep/28(VTQD_OPDHoldEnRel_flg)
  [VVMC_APSActive_flg] -> BOS/8(VVMC_APSActive_flg)
  [VTQD_VehActSpd_kph] -> DriverTqCoordination/20(VTQD_VehActSpd_kph)
  [VTQD_ActAPSPosn_pct] -> Creep/29(VTQD_ActAPSPosn_pct)
  [VTQD_APSReqTimer_s] -> DriverTqCoordination/21(VTQD_APSReqTimer_s)
  [VTQD_CreepEnable_flg] -> DriverTqCoordination/22(VTQD_CreepEnable_flg)
  [VTQD_OPDHoldEnRel_flg] -> PedalMapWhlTq/29(VTQD_OPDHoldEnRel_flg)
  [VINP_SASAngle_Deg] -> PedalMapWhlTq/30(VINP_SASAngle_Deg)
  [VINP_YawRate_degps] -> PedalMapWhlTq/31(VINP_YawRate_degps)
  [VVMC_ActStESCYaw_degps] -> PedalMapWhlTq/32(VVMC_ActStESCYaw_degps)
  VINP_SASAngle_Deg/1 -> [VINP_SASAngle_Deg]
  VINP_YawRate_degps/1 -> [VINP_YawRate_degps]
  VVMC_ActStESCYaw_degps/1 -> [VVMC_ActStESCYaw_degps]
  VVMC_CAASActive_flg/1 -> [VVMC_CAASActive_flg]
  [VVMC_CAASActive_flg] -> Creep/30(VVMC_CAASActive_flg)
  [VVMC_LongAcc_Gps] -> DriverTqCoordination/6(VVMC_LongAcc_Gps)
  [VTQD_APSReqTimer_s] -> PedalMapWhlTq/33(VTQD_APSReqTimer_s)
  [VTQD_LowIdleAccPedal_flg] -> BOS/9(VTQD_LowIdleAccPedal_flg)
  [VVMC_ACCOvrdMemTq_Nm] -> PedalMapWhlTq/34(VVMC_ACCOvrdMemTq_Nm)
  VVMC_ACCOvrdMemTq_Nm/1 -> [VVMC_ACCOvrdMemTq_Nm]
  VVMC_LastADASWhlTqReq_Nm/1 -> PedalMapWhlTq/35(VVMC_LastADASWhlTqReq_Nm)
  [VTQD_OPDHoldActRelTq_Nm] -> PedalMapWhlTq/36(VTQD_OPDHoldActRelTq_Nm)
  [VTQD_VehActSpd_kph] -> PedalMapWhlTq/37(VTQD_VehActSpd_kph)
  Creep/9(VTQD_HighBPSPosn_flg) -> [VTQD_HighBPSPosn_flg]
  [VTQD_HighBPSPosn_flg] -> BOS/10(VTQD_HighBPSPosn_flg)
  [VTQD_BrkSwSta_flg] -> BOS/11(VTQD_BrkSwSta_flg)
  VTQD_OPDHoldActRelTq_Nm/1 -> [VTQD_OPDHoldActRelTq_Nm]
  [VINP_IVISnowModeCmd_flg] -> PedalMapWhlTq/38(VINP_IVISnowModeCmd_flg)
  VINP_IVISnowModeCmd_flg/1 -> [VINP_IVISnowModeCmd_flg]
  [VDDM_EPB1CSErrCFS_flg] -> Creep/33(VDDM_EPB1CSErrCFS_flg)
  [VDDM_EPB1RCErrCFS_flg] -> Creep/32(VDDM_EPB1RCErrCFS_flg)
  [VDDM_EPBSigErrCFS_flg] -> Creep/34(VDDM_EPBSigErrCFS_flg)
  [VDDM_EPB1NoComCFS_flg] -> Creep/31(VDDM_EPB1NoComCFS_flg)
  VDDM_EPB1CSErrCFS_flg/1 -> [VDDM_EPB1CSErrCFS_flg]
  VDDM_EPBSigErrCFS_flg/1 -> [VDDM_EPBSigErrCFS_flg]
  VDDM_EPB1NoComCFS_flg/1 -> [VDDM_EPB1NoComCFS_flg]
  VDDM_EPB1RCErrCFS_flg/1 -> [VDDM_EPB1RCErrCFS_flg]

== system tqd/TQD/TorqueDemand/TorqueModule/ExtTqFuncHandShaking ==
  VPMM_PwrSta_enum : Inport
  VTQD_MCUReady4Ext_flg : Inport  Port=2
  VINP_HVBattErr_flg : Inport  Port=3
  VINP_DCDCFaultSta_enum : Inport  Port=4
  VINP_EPBErrSta_enum : Inport  Port=5
  VINP_DrDoorSW_flg : Inport  Port=6
  VINP_PsDoorSW_flg : Inport  Port=7
  VINP_RRDoorSW_flg : Inport  Port=8
  VINP_RLDoorSW_flg : Inport  Port=9
  VINP_HoodSW_flg : Inport  Port=10
  VINP_TailgateSW_flg : Inport  Port=11
  VVMC_APSActive_flg : Inport  Port=12
  Constant1 : Constant  Value=KTQD_ExtTqAllow_flg_ovrdflg
  Constant10 : Constant  Value=TRUE
  Constant11 : Constant  Value=FALSE
  Constant12 : Constant  Value=KTQD_PassAPSActive_flg_ovrdflg
  Constant13 : Constant  Value=KTQD_ExtDoorAllow_flg_ovrdflg
  Constant14 : Constant  Value=KTQD_ExtDoorAllow_flg_ovrdval
  Constant15 : Constant  Value=ENUM_POWERSTA_READY
  Constant16 : Constant  Value=ENUM_POWERSTA_ON
  Constant17 : Constant  Value=ENUM_POWERSTA_READY
  Constant18 : Constant  Value=ENUM_POWERSTA_ON
  Constant19 : Constant  Value=KTQD_PassAPSActive_flg_ovrdflg
  Constant2 : Constant  Value=ENUM_DCDCFAULTSTA_WORKING
  Constant20 : Constant  Value=KTQD_PassAPSActive_flg_ovrdval
  Constant21 : Constant  Value=KTQD_PassAPSActive_flg_ovrdval
  Constant3 : Constant  Value=KTQD_ExtTqAllow_flg_ovrdval
  Constant4 : Constant  Value=ENUM_DCDCFAULTSTA_WORKING
  Constant5 : Constant  Value=ENUM_EPBERROR_NORMAL
  Constant6 : Constant  Value=KTQD_ExtShftAllow_flg_ovrdflg
  Constant7 : Constant  Value=KTQD_ExtShftAllow_flg_ovrdval
  Constant8 : Constant  Value=TRUE
  Constant9 : Constant  Value=FALSE
  Equal{1..3,5..8} (7 alike) : RelationalOperator  Operator===  OutDataTypeStr=boolean  RndMeth=Simplest
  LiuzgSwitch{1..7} (7 alike) : Switch  Criteria=u2 ~= 0
      settings: AttributesFormatString=<%<Criteria>>
  Logical Operator : Logic  Operator=NOT  AllPortsSameDT=off  OutDataTypeStr=boolean
  Logical Operator1 : Logic  Operator=NOT  AllPortsSameDT=off  OutDataTypeStr=boolean
  Logical Operator2 : Logic  Operator=OR  AllPortsSameDT=off  OutDataTypeStr=boolean
  Logical Operator3 : Logic  Operator=OR  AllPortsSameDT=off  OutDataTypeStr=boolean
  Logical Operator4 : Logic  AllPortsSameDT=off  OutDataTypeStr=boolean
  Logical Operator5 : Logic  AllPortsSameDT=off  OutDataTypeStr=boolean
  NOT{,1..5} (6 alike) : Logic  Operator=NOT  AllPortsSameDT=off  OutDataTypeStr=boolean
  OR : Logic  Inputs=4  AllPortsSameDT=off  OutDataTypeStr=boolean
  OR1 : Logic  Inputs=5  AllPortsSameDT=off  OutDataTypeStr=boolean
  OR2 : Logic  Inputs=6  AllPortsSameDT=off  OutDataTypeStr=boolean
  VTQD_ExternalTqAllow_flg : Outport
  VTQD_ExtShftAllow_flg : Outport  Port=2
  VTQD_ExtDoorAllow_flg : Outport  Port=3
  wires:
  Logical Operator/1 -> OR/2
  VTQD_MCUReady4Ext_flg/1 -> [VTQD_MCUReady4Ext_flg]
  Constant2/1 -> Equal2/2
  [VINP_DCDCFaultSta_enum] -> Equal2/1
  [VTQD_MCUReady4Ext_flg] -> OR/4
  [VINP_HVBattErr_flg] -> Logical Operator/1
  Equal2/1 -> OR/3
  VINP_HVBattErr_flg/1 -> [VINP_HVBattErr_flg]
  VINP_DCDCFaultSta_enum/1 -> [VINP_DCDCFaultSta_enum]
  VPMM_PwrSta_enum/1 -> [VPMM_PwrSta_enum]
  LiuzgSwitch1/1 -> VTQD_ExternalTqAllow_flg/1  "VTQD_ExternalTqAllow_flg"
  Constant1/1 -> LiuzgSwitch1/2
  Constant3/1 -> LiuzgSwitch1/1
  VINP_EPBErrSta_enum/1 -> [VINP_EPBErrSta_enum]
  Constant5/1 -> Equal3/2
  LiuzgSwitch2/1 -> VTQD_ExtShftAllow_flg/1  "VTQD_ExtShftAllow_flg"
  Constant4/1 -> Equal1/2
  [VINP_HVBattErr_flg] -> Logical Operator1/1
  [VTQD_MCUReady4Ext_flg] -> OR1/5
  [VINP_EPBErrSta_enum] -> Equal3/1
  Equal1/1 -> OR1/3
  Equal3/1 -> OR1/2
  Logical Operator1/1 -> OR1/4
  [VINP_DCDCFaultSta_enum] -> Equal1/1
  Constant6/1 -> LiuzgSwitch2/2
  Constant7/1 -> LiuzgSwitch2/1
  OR1/1 -> LiuzgSwitch3/2
  Constant8/1 -> LiuzgSwitch3/1
  Constant9/1 -> LiuzgSwitch3/3
  Constant11/1 -> LiuzgSwitch4/3
  Constant10/1 -> LiuzgSwitch4/1
  OR/1 -> LiuzgSwitch4/2
  LiuzgSwitch5/1 -> VTQD_ExtDoorAllow_flg/1  "VTQD_ExtDoorAllow_flg"
  Constant14/1 -> LiuzgSwitch5/1
  Constant13/1 -> LiuzgSwitch5/2
  NOT5/1 -> OR2/6
  NOT4/1 -> OR2/5
  OR2/1 -> LiuzgSwitch5/3
  NOT2/1 -> OR2/3
  NOT/1 -> OR2/1
  NOT1/1 -> OR2/2
  NOT3/1 -> OR2/4
  [VINP_DrDoorSW_flg] -> NOT/1
  VINP_TailgateSW_flg/1 -> [VINP_TailgateSW_flg]
  VINP_RRDoorSW_flg/1 -> [VINP_RRDoorSW_flg]
  VINP_RLDoorSW_flg/1 -> [VINP_RLDoorSW_flg]
  VINP_HoodSW_flg/1 -> [VINP_HoodSW_flg]
  VINP_DrDoorSW_flg/1 -> [VINP_DrDoorSW_flg]
  VINP_PsDoorSW_flg/1 -> [VINP_PsDoorSW_flg]
  [VINP_PsDoorSW_flg] -> NOT1/1
  [VINP_RRDoorSW_flg] -> NOT2/1
  [VINP_RLDoorSW_flg] -> NOT3/1
  [VINP_HoodSW_flg] -> NOT4/1
  [VINP_TailgateSW_flg] -> NOT5/1
  [VPMM_PwrSta_enum] -> Equal5/1
  Constant15/1 -> Equal5/2
  [VPMM_PwrSta_enum] -> Equal6/1
  Constant16/1 -> Equal6/2
  Equal5/1 -> Logical Operator2/1
  Equal6/1 -> Logical Operator2/2
  Logical Operator2/1 -> OR1/1
  Equal8/1 -> Logical Operator3/2
  Equal7/1 -> Logical Operator3/1
  [VPMM_PwrSta_enum] -> Equal8/1
  Constant17/1 -> Equal7/2
  [VPMM_PwrSta_enum] -> Equal7/1
  Logical Operator3/1 -> OR/1
  Constant18/1 -> Equal8/2
  Logical Operator4/1 -> LiuzgSwitch6/2
  [VVMC_APSActive_flg] -> Logical Operator4/1
  LiuzgSwitch4/1 -> LiuzgSwitch6/3
  Constant19/1 -> Logical Operator4/2
  Constant21/1 -> LiuzgSwitch6/1
  LiuzgSwitch6/1 -> LiuzgSwitch1/3
  Logical Operator5/1 -> LiuzgSwitch7/2
  Constant12/1 -> Logical Operator5/2
  LiuzgSwitch3/1 -> LiuzgSwitch7/3
  Constant20/1 -> LiuzgSwitch7/1
  [VVMC_APSActive_flg] -> Logical Operator5/1
  LiuzgSwitch7/1 -> LiuzgSwitch2/3
  VVMC_APSActive_flg/1 -> [VVMC_APSActive_flg]

== system tqd/TQD/TorqueDemand/TorqueModule/OPD Hold ==
  task_time_s : Inport
  VTQD_RegenMode_enum : Inport  Port=2
  VTQD_GearActualPosn_enum : Inport  Port=3
  VTQD_VehActSpd_kph : Inport  Port=4
  VTQD_ActBPSPosn_pct : Inport  Port=5
  VVMC_ADASActive_flg : Inport  Port=6
  VVMC_CruzActive_flg : Inport  Port=7
  VTQD_ParkRequest_flg : Inport  Port=8
  VVMC_EstSlope_Deg : Inport  Port=9
  VVMC_LongAcc_Gps : Inport  Port=10
  VTQD_AntiBlockRrActDisTime_s : Inport  Port=11
  VTQD_RrAntiBlockAactive_flg : Inport  Port=12
  VTQD_AntiBlockFrActDisTime_s : Inport  Port=13
  VTQD_FrAntiBlockAactive_flg : Inport  Port=14
  VTQR_NoABSFEDUWhlTqReq_Nm : Inport  Port=15
  VTQR_NoABSREDUWhlTqReq_Nm : Inport  Port=16
  VINP_EPBSta_enum : Inport  Port=17
  VPMM_PwrSta_enum : Inport  Port=18
  VTQD_LowIdleAccPedal_flg : Inport  Port=19
  VTQD_ActAPSPosn_pct : Inport  Port=20
  VTQD_FrOPDHoldRelTqGain_Nm : Inport  Port=21
  VTQD_RrOPDHoldRelTqGain_Nm : Inport  Port=22
  VINP_FrPTCSActive_flg : Inport  Port=23
  VINP_RrPTCSActive_flg : Inport  Port=24
  VINP_ESCActive_flg : Inport  Port=25
  VINP_ABSActive_flg : Inport  Port=26
  VVMC_APSActive_flg : Inport  Port=27
  Deceleration Calculation : Subsystem
  "OPDHold Request " : Subsystem
  Parking Requeest Backup : Subsystem
  Release Condition : Subsystem
  System Status : Subsystem
  VTQD_APSStaSys_enum : Outport
  VTQD_APSReq_enum : Outport  Port=2
  VTQD_APSDecReqA_flg : Outport  Port=3
  VTQD_APSDecReq_mps2 : Outport  Port=4
  VTQD_ActParkRequest_flg : Outport  Port=5
  VTQD_APSReqTimer_s : Outport  Port=6
  VTQD_OPDHoldEnRel_flg : Outport  Port=7
  VTQD_OPDHoldDelayForP_flg : Outport  Port=8
  VTQD_OPDHoldAllowPark_flg : Outport  Port=9
  VTQD_OPDHoldLamp_flg : Outport  Port=10
  VTQD_OPDHoldActRelTq_Nm : Outport  Port=11
  wires:
  VTQD_RegenMode_enum/1 -> [VTQD_RegenMode_enum]
  VTQD_GearActualPosn_enum/1 -> [VTQD_GearActualPosn_enum]
  VTQD_VehActSpd_kph/1 -> [VTQD_VehActSpd_kph]
  task_time_s/1 -> [task_time_s]
  [VTQD_APSStaSys_enum] -> VTQD_APSStaSys_enum/1
  [VTQD_APSReq_enum] -> VTQD_APSReq_enum/1
  [VTQD_APSDecReq_mps2] -> VTQD_APSDecReq_mps2/1
  [VTQD_APSDecReqA_flg] -> VTQD_APSDecReqA_flg/1
  VTQD_ActBPSPosn_pct/1 -> [VTQD_ActBPSPosn_pct]
  VVMC_ADASActive_flg/1 -> [VVMC_ADASActive_flg]
  VVMC_CruzActive_flg/1 -> [VVMC_CruzActive_flg]
  [VTQD_ActParkRequest_flg] -> VTQD_ActParkRequest_flg/1
  VTQD_ParkRequest_flg/1 -> [VTQD_ParkRequest_flg]
  VVMC_EstSlope_Deg/1 -> [VVMC_EstSlope_Deg]
  VVMC_LongAcc_Gps/1 -> [VVMC_LongAcc_Gps]
  VTQD_FrAntiBlockAactive_flg/1 -> [VTQD_FrAntiBlockAactive_flg]
  VTQD_AntiBlockFrActDisTime_s/1 -> [VTQD_AntiBlockFrActDisTime_s]
  VTQD_RrAntiBlockAactive_flg/1 -> [VTQD_RrAntiBlockAactive_flg]
  VTQD_AntiBlockRrActDisTime_s/1 -> [VTQD_AntiBlockRrActDisTime_s]
  VTQR_NoABSFEDUWhlTqReq_Nm/1 -> [VTQR_NoABSFEDUWhlTqReq_Nm]
  VTQR_NoABSREDUWhlTqReq_Nm/1 -> [VTQR_NoABSREDUWhlTqReq_Nm]
  VINP_EPBSta_enum/1 -> [VINP_EPBSta_enum]
  VPMM_PwrSta_enum/1 -> [VPMM_PwrSta_enum]
  [VTQD_OPDHoldDelayForP_flg] -> VTQD_OPDHoldDelayForP_flg/1
  [VTQD_APSReqTimer_s] -> VTQD_APSReqTimer_s/1
  [VTQD_OPDHoldEnRel_flg] -> VTQD_OPDHoldEnRel_flg/1
  [VTQD_AutoHoldRelease_flg] -> System Status/4(VTQD_AutiHoldRelease_flg)
  System Status/1(VTQD_APSStaSys_enum) -> [VTQD_APSStaSys_enum]
  [VTQD_ActBPSPosn_pct] -> Release Condition/5(VTQD_ActBPSPosn_pct)
  [VTQD_VehActSpd_kph] -> Release Condition/2(VTQD_VehActSpd_kph)
  Release Condition/1(VTQD_AutoHoldRelease_flg) -> [VTQD_AutoHoldRelease_flg]
  Release Condition/2(VTQD_OPDHoldEnRel_flg) -> [VTQD_OPDHoldEnRel_flg]
  System Status/2(VTQD_OPDHoldDelayForP_flg) -> [VTQD_OPDHoldDelayForP_flg]
  [VTQD_VehActSpd_kph] -> "OPDHold Request "/1(VTQD_VehActSpd_kph)
  [VTQD_APSStaSys_enum] -> "OPDHold Request "/2(VTQD_APSStaSys_enum)
  [VTQD_AutoHoldRelease_flg] -> "OPDHold Request "/3(VTQD_AutiHoldRelease_flg)
  [task_time_s] -> "OPDHold Request "/4(task_time_s)
  "OPDHold Request "/1(VTQD_APSReqTimer_s) -> [VTQD_APSReqTimer_s]
  "OPDHold Request "/2(VTQD_APSReq_enum) -> [VTQD_APSReq_enum]
  "OPDHold Request "/3(VTQD_APSDecReqA_flg) -> [VTQD_APSDecReqA_flg]
  [VTQD_VehActSpd_kph] -> Deceleration Calculation/1(VTQD_VehActSpd_kph)
  [VTQD_APSReqTimer_s] -> Deceleration Calculation/3(VTQD_APSReqTimer_s)
  [VVMC_EstSlope_Deg] -> Deceleration Calculation/4(VVMC_EstSlope_Deg)
  [VTQD_APSDecReqA_flg] -> Deceleration Calculation/5(VTQD_APSDecReqA_flg)
  Deceleration Calculation/1(VTQD_APSDecReq_mps2) -> [VTQD_APSDecReq_mps2]
  [VTQD_APSReq_enum] -> Parking Requeest Backup/1(VTQD_APSReq_enum)
  [VTQD_APSReqTimer_s] -> Parking Requeest Backup/2(VTQD_APSReqTimer_s)
  Parking Requeest Backup/1(VTQD_ActParkRequest_flg) -> [VTQD_ActParkRequest_flg]
  [VTQD_GearActualPosn_enum] -> System Status/1(VTQD_GearActualPosn_enum)
  [VINP_EPBSta_enum] -> System Status/2(VINP_EPBSta_enum)
  [VTQD_RegenMode_enum] -> System Status/3(VTQD_RegenMode_enum)
  [VTQD_AntiBlockRrActDisTime_s] -> System Status/5(VTQD_AntiBlockRrActDisTime_s)
  [VTQD_RrAntiBlockAactive_flg] -> System Status/6(VTQD_RrAntiBlockAactive_flg)
  [VTQD_ActBPSPosn_pct] -> System Status/7(VTQD_ActBPSPosn_pct)
  [VTQD_AntiBlockFrActDisTime_s] -> System Status/8(VTQD_AntiBlockFrActDisTime_s)
  [VTQD_FrAntiBlockAactive_flg] -> System Status/9(VTQD_FrAntiBlockAactive_flg)
  [VVMC_ADASActive_flg] -> System Status/10(VVMC_ADASActive_flg)
  [VPMM_PwrSta_enum] -> System Status/11(VPMM_PwrSta_enum)
  [VVMC_CruzActive_flg] -> System Status/12(VVMC_CruzActive_flg)
  [VTQD_VehActSpd_kph] -> System Status/13(VTQD_VehActSpd_kph)
  [VVMC_EstSlope_Deg] -> Release Condition/1(VVMC_EstSlope_Deg)
  [VTQR_NoABSFEDUWhlTqReq_Nm] -> Release Condition/3(VTQR_NoABSFEDUWhlTqReq_Nm)
  [VTQR_NoABSREDUWhlTqReq_Nm] -> Release Condition/4(VTQR_NoABSREDUWhlTqReq_Nm)
  [task_time_s] -> Release Condition/6(task_time_s)
  [VVMC_LongAcc_Gps] -> Deceleration Calculation/2(VVMC_LongAcc_Gps)
  [VTQD_ParkRequest_flg] -> Parking Requeest Backup/3(VTQD_ParkRequest_flg)
  [VTQD_AutoHoldRelease_flg] -> Deceleration Calculation/6(VTQD_AutiHoldRelease_flg)
  [VVMC_EstSlope_Deg] -> "OPDHold Request "/5(VVMC_EstSlope_Deg)
  [VTQD_APSReqTimer_s] -> Release Condition/7(VTQD_APSReqTimer_s)
  [VTQD_LowIdleAccPedal_flg] -> Release Condition/8(VTQD_LowIdleAccPedal_flg)
  VTQD_LowIdleAccPedal_flg/1 -> [VTQD_LowIdleAccPedal_flg]
  System Status/3(VTQD_OPDHoldRgnOn2Off_flg) -> [VTQD_OPDHoldRgnOn2Off_flg]
  [VTQD_OPDHoldRgnOn2Off_flg] -> Release Condition/9(VTQD_OPDHoldRgnOn2Off_flg)
  [task_time_s] -> Parking Requeest Backup/4(task_time_s)
  [VTQD_AutoHoldRelease_flg] -> Parking Requeest Backup/5(VTQD_AutiHoldRelease_flg)
  [task_time_s] -> Deceleration Calculation/7(task_time_s)
  [VTQD_ActAPSPosn_pct] -> Deceleration Calculation/8(VTQD_ActAPSPosn_pct)
  VTQD_ActAPSPosn_pct/1 -> [VTQD_ActAPSPosn_pct]
  Parking Requeest Backup/2(VTQD_OPDHoldAllowPark_flg) -> [VTQD_OPDHoldAllowPark_flg]
  [VTQD_OPDHoldAllowPark_flg] -> VTQD_OPDHoldAllowPark_flg/1
  [VTQD_ActAPSPosn_pct] -> Release Condition/10(VTQD_ActAPSPosn_pct)
  VTQD_RrOPDHoldRelTqGain_Nm/1 -> [VTQD_RrOPDHoldRelTqGain_Nm]
  VTQD_FrOPDHoldRelTqGain_Nm/1 -> [VTQD_FrOPDHoldRelTqGain_Nm]
  [VTQD_RrOPDHoldRelTqGain_Nm] -> Release Condition/12(VTQD_RrOPDHoldRelTqGain_Nm)
  [VTQD_FrOPDHoldRelTqGain_Nm] -> Release Condition/11(VTQD_FrOPDHoldRelTqGain_Nm)
  "OPDHold Request "/4(VTQD_OPDHoldLamp_flg) -> [VTQD_OPDHoldLamp_flg]
  [VTQD_OPDHoldLamp_flg] -> VTQD_OPDHoldLamp_flg/1
  [VTQD_OPDHoldActRelTq_Nm] -> VTQD_OPDHoldActRelTq_Nm/1
  Release Condition/3(VTQD_OPDHoldActRelTq_Nm) -> [VTQD_OPDHoldActRelTq_Nm]
  [VINP_ABSActive_flg] -> System Status/19(VINP_ABSActive_flg)
  [VVMC_EstSlope_Deg] -> System Status/14(VVMC_EstSlope_Deg)
  [task_time_s] -> System Status/15(task_time_s)
  [VINP_ESCActive_flg] -> System Status/18(VINP_ESCActive_flg)
  [VINP_FrPTCSActive_flg] -> System Status/16(VINP_FrPTCSActive_flg)
  [VINP_RrPTCSActive_flg] -> System Status/17(VINP_RrPTCSActive_flg)
  VINP_FrPTCSActive_flg/1 -> [VINP_FrPTCSActive_flg]
  VINP_RrPTCSActive_flg/1 -> [VINP_RrPTCSActive_flg]
  VINP_ESCActive_flg/1 -> [VINP_ESCActive_flg]
  VINP_ABSActive_flg/1 -> [VINP_ABSActive_flg]
  [VVMC_APSActive_flg] -> System Status/20(VVMC_APSActive_flg)
  VVMC_APSActive_flg/1 -> [VVMC_APSActive_flg]
